simulink model "code"  (R2023a)
settings: Solver=FixedStepAuto  StartTime=0.0  StopTime=inf  FixedStep=0.01  RelTol=1e-3  EnableMultiTasking=on
values from neighbouring files (symbols this model uses):
  K = lqr(A, B(:,1), Q, R)    [controller.m]
libraries: simulink x2, arduinolib x1
settings Model: ExtModeTrigDuration=2  Creator=husse  LastModifiedBy=mahmoudyassermahmoud
settings SolverCC: AlgebraicLoopSolver=TrustRegion  AutoInsertRateTranBlk=on
settings OptimizationCC: EnhancedBackFolding=on  PassReuseOutputArgsThreshold=0  MaxStackSize=64  OptimizeBlockOrder=speed  DifferentSizesBufferReuse=on  OptimizationCustomize=off
settings DebuggingCC: ParameterTunabilityLossMsg=error
settings HardwareCC: ProdBitPerPointer=32  ProdBitPerSizeT=32  ProdBitPerPtrDiffT=32  ProdLargestAtomicInteger=Long  ProdLargestAtomicFloat=Double  ProdWordSize=32  ProdHWDeviceType=ARM Compatible->ARM Cortex
settings SFSimCC: MATLABDynamicMemAlloc=off
settings RTWCC: Description=Embedded Coder  SystemTargetFile=ert.tlc  HardwareBoard=ESP32-WROOM(Arduino Compatible)  TLCOptions="-aInlineSetEventsForThisBaseRateFcn=TLC_FALSE -aSuppressMultiTaskScheduler=TLC_FALSE    -aRateBasedStepFcn=0"  TemplateMakefile=ert_default_tmf  Toolchain=ESP32  BuildConfiguration=Faster Runs
settings CodeAppCC: ForceParamTrailComments=on  OperatorAnnotations=on
settings ERTTargetCC: ERTCustomFileBanners=off  SupportContinuousTime=on  SupportNonInlinedSFcns=on  RemoveResetFunc=off  SupportVariableSizeSignals=on  ModelStepFunctionPrototypeControlCompliant=off  ExtModeTransport=3  ExtModeStaticAlloc=on  ExtModeAutomaticAllocSize=off  ExtModeStaticAllocSize=65536  ExtModeMexFile=ext_xcp  ExtModeIntrfLevel=Level2 - Open

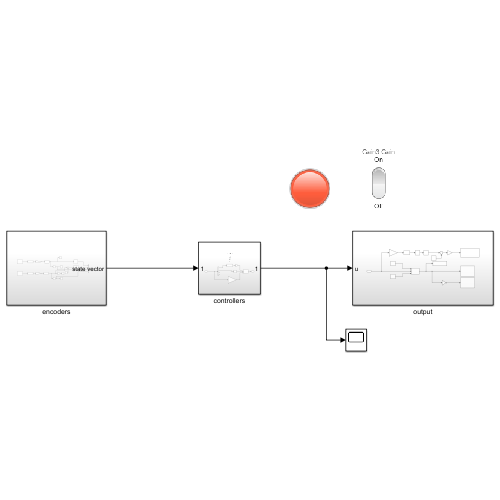
[thumbnail: Simulink's stored preview of the top-level diagram]
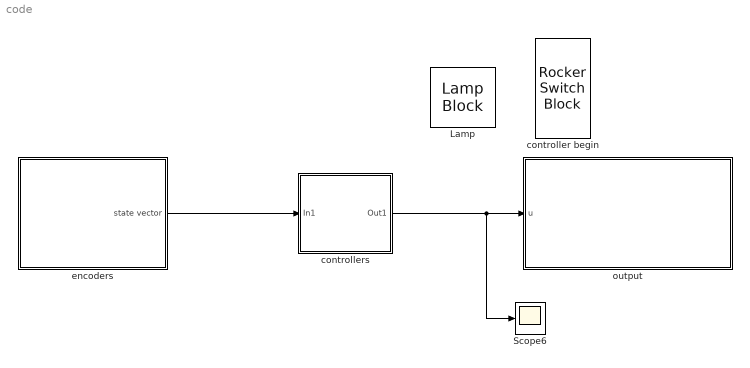
== system code ==
  Lamp : LampBlock  LabelPosition=Hide
  Scope6 : Scope
  controller begin : RockerSwitchBlock
      settings: Values={{'Off', 'On'}, [0 1]}
  controllers : Subsystem
  encoders : Subsystem
  output : Subsystem
  wires:
  controllers/1(Out1) -> Scope6/1, output/1(u)
  encoders/1(state vector) -> controllers/1(In1)

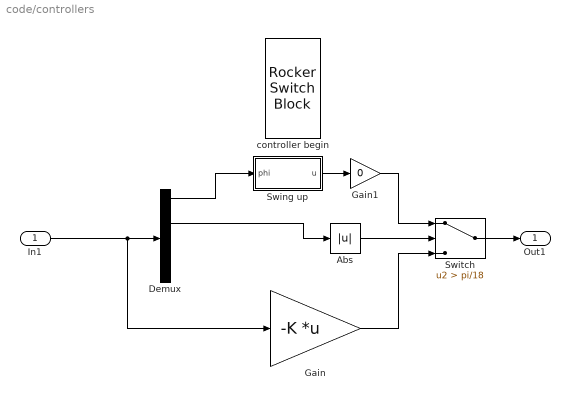
== system code/controllers ==
  In1 : Inport
  Abs : Abs  SaturateOnIntegerOverflow=off
  Demux : Demux
  Gain : Gain  Gain=-K  Multiplication=Matrix(K*u) (u vector)
  Gain1 : Gain  Gain=0
  Swing up : Subsystem
  Switch : Switch  Criteria=u2 > Threshold  Threshold=pi/18  SaturateOnIntegerOverflow=off  InputSameDT=off
  controller begin : RockerSwitchBlock
      settings: Values={{'Off', 'On'}, [0 1]}
  Out1 : Outport
  wires:
  In1/1 -> Demux/1, Gain/1
  Switch/1 -> Out1/1
  Demux/2 -> Abs/1
  Abs/1 -> Switch/2
  Gain/1 -> Switch/3
  Demux/1 -> Swing up/1(phi)
  Swing up/1(u) -> Gain1/1
  Gain1/1 -> Switch/1

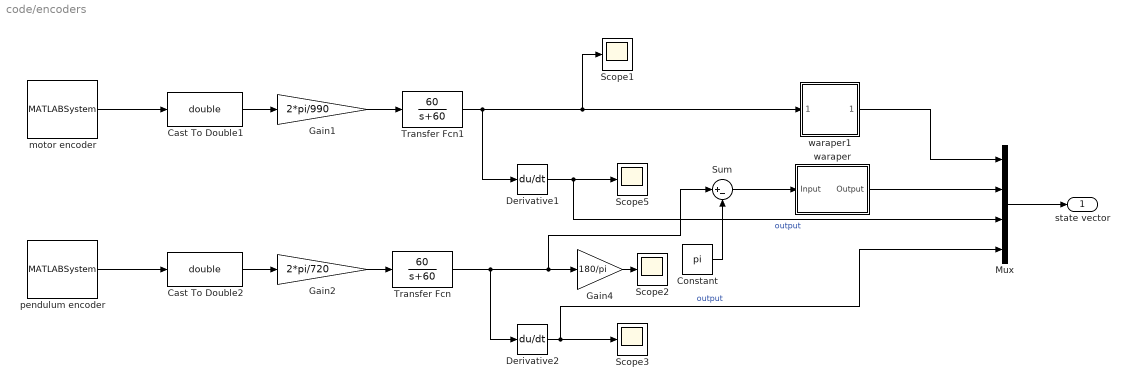
== system code/encoders ==
  Cast To Double1 : DataTypeConversion  OutDataTypeStr=double  SaturateOnIntegerOverflow=off  RndMeth=Floor
  Cast To Double2 : DataTypeConversion  OutDataTypeStr=double  SaturateOnIntegerOverflow=off  RndMeth=Floor
  Constant : Constant  Value=pi
  Derivative1 : Derivative
  Derivative2 : Derivative
  Gain1 : Gain  Gain=2*pi/990
  Gain2 : Gain  Gain=2*pi/720
  Gain4 : Gain  Gain=180/pi
  Mux : Mux
  Scope{1..3,5} (4 alike) : Scope
  Sum : Sum  Inputs=|+-
  Transfer Fcn : TransferFcn  Numerator=[60]  Denominator=[1 60]
  Transfer Fcn1 : TransferFcn  Numerator=[60]  Denominator=[1 60]
  motor encoder : MATLABSystem  System=Encoder_esp32  Encoder=0  PinA=18  PinB=19  SampleTime=0.01
      mask Type: Encoder_esp32
      mask Display:
      | disp('Encoder');
      | port_label('output',1,'y');
  pendulum encoder : MATLABSystem  System=Encoder_esp32  Encoder=1  PinA=22  PinB=23  SampleTime=0.01
      mask Type: Encoder_esp32
      mask Display:
      | disp('Encoder');
      | port_label('output',1,'y');
  waraper : Subsystem
  waraper1 : Subsystem
  state vector : Outport
  wires:
  Derivative2/1 -> Scope3/1, Mux/4  "output"
  Cast To Double1/1 -> Gain1/1
  pendulum encoder/1 -> Cast To Double2/1
  Derivative1/1 -> Mux/3, Scope5/1  "output"
  motor encoder/1 -> Cast To Double1/1
  Cast To Double2/1 -> Gain2/1
  Constant/1 -> Sum/2
  Sum/1 -> waraper/1(Input)
  Gain4/1 -> Scope2/1
  Mux/1 -> state vector/1
  Gain2/1 -> Transfer Fcn/1
  Gain1/1 -> Transfer Fcn1/1
  Transfer Fcn/1 -> Sum/1, Gain4/1, Derivative2/1
  Transfer Fcn1/1 -> Scope1/1, waraper1/1(Input), Derivative1/1
  waraper/1(Output) -> Mux/2
  waraper1/1(Output) -> Mux/1

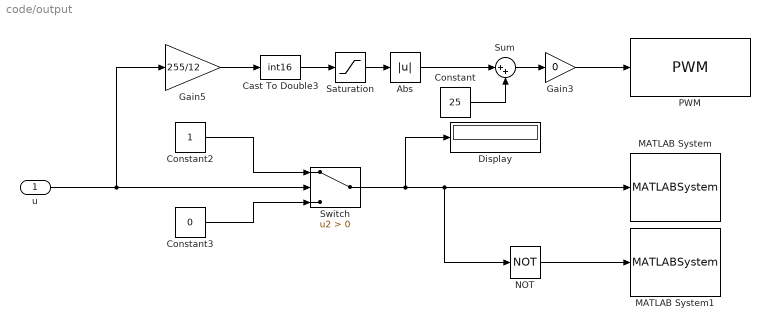
== system code/output ==
  u : Inport
  Abs : Abs  SaturateOnIntegerOverflow=off
  Cast To Double3 : DataTypeConversion  OutDataTypeStr=int16  SaturateOnIntegerOverflow=off  RndMeth=Floor
  Constant : Constant  Value=25
  Constant2 : Constant
  Constant3 : Constant  Value=0
  Display : Display
  Gain3 : Gain  Gain=0
  Gain5 : Gain  Gain=255/12
  MATLAB System : MATLABSystem  System=DigitalWrite_arduino  Pin=5
      mask Type: DigitalWrite_arduino
      mask Display:
      | disp('Digital Write');
      | port_label('input',1,'u');
  MATLAB System1 : MATLABSystem  System=DigitalWrite_arduino  Pin=4
      mask Type: DigitalWrite_arduino
      mask Display:
      | disp('Digital Write');
      | port_label('input',1,'u');
  NOT : Logic  Operator=NOT  IconShape=distinctive  AllPortsSameDT=off  OutDataTypeStr=boolean
  PWM : arduinolib/PWM  pinNumber=21  frequencyType=Default  desiredFrequency=490.2  achievableFrequency=490.2
  Saturation : Saturate  UpperLimit=255  LowerLimit=-255
  Sum : Sum  Inputs=|++
  Switch : Switch  Criteria=u2 > Threshold  SaturateOnIntegerOverflow=off  InputSameDT=off
  wires:
  Switch/1 -> Display/1, NOT/1, MATLAB System/1
  Saturation/1 -> Abs/1
  u/1 -> Gain5/1, Switch/2
  Constant2/1 -> Switch/1
  Cast To Double3/1 -> Saturation/1
  Constant3/1 -> Switch/3
  Gain5/1 -> Cast To Double3/1
  NOT/1 -> MATLAB System1/1
  Gain3/1 -> PWM/1
  Abs/1 -> Sum/1
  Sum/1 -> Gain3/1
  Constant/1 -> Sum/2

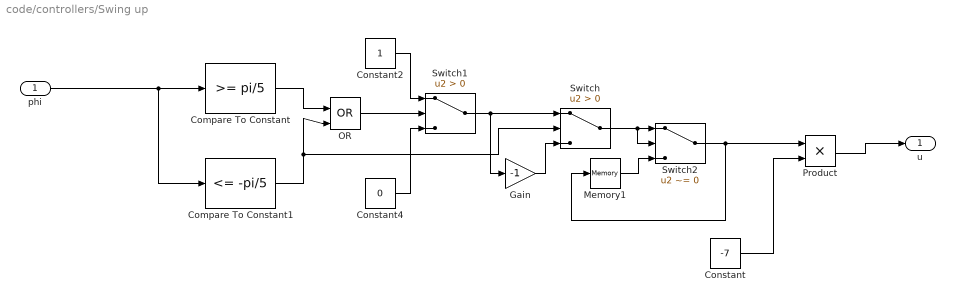
== system code/controllers/Swing up ==
  phi : Inport
  Compare To Constant : simulink/Logic and Bit Operations/Compare To Constant  relop=>=  const=pi/5  OutDataTypeStr=boolean
  Compare To Constant1 : simulink/Logic and Bit Operations/Compare To Constant  relop=<=  const=-pi/5  OutDataTypeStr=boolean
  Constant : Constant  Value=-7
  Constant2 : Constant
  Constant4 : Constant  Value=0
  Gain : Gain  Gain=-1
  Memory1 : Memory  InitialCondition=1
  OR : Logic  Operator=OR  IconShape=distinctive  AllPortsSameDT=off  OutDataTypeStr=boolean
  Product : Product
  Switch : Switch  Criteria=u2 > Threshold  SaturateOnIntegerOverflow=off  InputSameDT=off
  Switch1 : Switch  Criteria=u2 > Threshold  SaturateOnIntegerOverflow=off  InputSameDT=off
  Switch2 : Switch  Criteria=u2 ~= 0  SaturateOnIntegerOverflow=off  InputSameDT=off
  u : Outport
  wires:
  Switch1/1 -> Gain/1, Switch/1
  phi/1 -> Compare To Constant1/1, Compare To Constant/1
  Constant4/1 -> Switch1/3
  Constant2/1 -> Switch1/1
  Compare To Constant1/1 -> Switch/2, OR/2
  Compare To Constant/1 -> OR/1
  Gain/1 -> Switch/3
  OR/1 -> Switch1/2
  Constant/1 -> Product/2
  Switch/1 -> Switch2/2, Switch2/1
  Product/1 -> u/1
  Switch2/1 -> Product/1, Memory1/1
  Memory1/1 -> Switch2/3

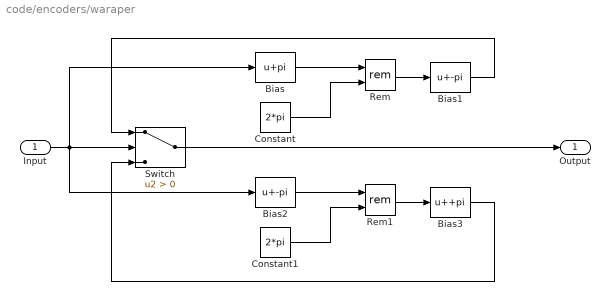
== system code/encoders/waraper ==
  Input : Inport
  Bias : Bias  Bias=pi  SaturateOnIntegerOverflow=off
  Bias1 : Bias  Bias=-pi  SaturateOnIntegerOverflow=off
  Bias2 : Bias  Bias=-pi  SaturateOnIntegerOverflow=off
  Bias3 : Bias  Bias=+pi  SaturateOnIntegerOverflow=off
  Constant : Constant  Value=2*pi
  Constant1 : Constant  Value=2*pi
  Rem : Math  Operator=rem
  Rem1 : Math  Operator=rem
  Switch : Switch  Criteria=u2 > Threshold  SaturateOnIntegerOverflow=off  InputSameDT=off
  Output : Outport
  wires:
  Constant/1 -> Rem/2
  Bias/1 -> Rem/1
  Input/1 -> Bias/1, Bias2/1, Switch/2
  Bias3/1 -> Switch/3
  Bias2/1 -> Rem1/1
  Rem1/1 -> Bias3/1
  Constant1/1 -> Rem1/2
  Switch/1 -> Output/1
  Rem/1 -> Bias1/1
  Bias1/1 -> Switch/1

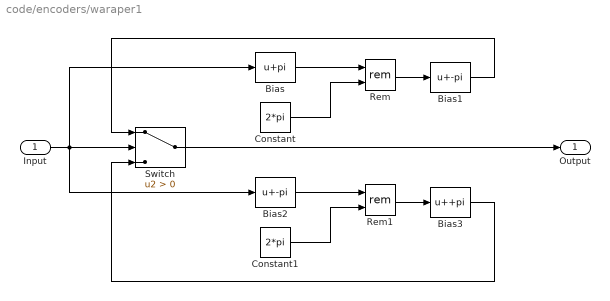
== system code/encoders/waraper1 ==
  Input : Inport
  Bias : Bias  Bias=pi  SaturateOnIntegerOverflow=off
  Bias1 : Bias  Bias=-pi  SaturateOnIntegerOverflow=off
  Bias2 : Bias  Bias=-pi  SaturateOnIntegerOverflow=off
  Bias3 : Bias  Bias=+pi  SaturateOnIntegerOverflow=off
  Constant : Constant  Value=2*pi
  Constant1 : Constant  Value=2*pi
  Rem : Math  Operator=rem
  Rem1 : Math  Operator=rem
  Switch : Switch  Criteria=u2 > Threshold  SaturateOnIntegerOverflow=off  InputSameDT=off
  Output : Outport
  wires:
  Constant/1 -> Rem/2
  Bias/1 -> Rem/1
  Input/1 -> Bias/1, Bias2/1, Switch/2
  Bias3/1 -> Switch/3
  Bias2/1 -> Rem1/1
  Rem1/1 -> Bias3/1
  Constant1/1 -> Rem1/2
  Switch/1 -> Output/1
  Rem/1 -> Bias1/1
  Bias1/1 -> Switch/1
